simulink model "AA"  (R2021b)
settings: Solver=VariableStepAuto  StartTime=0.0  StopTime=50  RelTol=1e-3
values from neighbouring files (symbols this model uses):
  A = [ybb  yp+w0/u0 yr-1 g*ctt0/u0 ... (first row only)    [main.m]
  B = [0    ydr ... (first row only)    [main.m]
undefined symbols (not defined in the file or in its folder): C, D
settings Model: Creator=User  LastModifiedBy=User

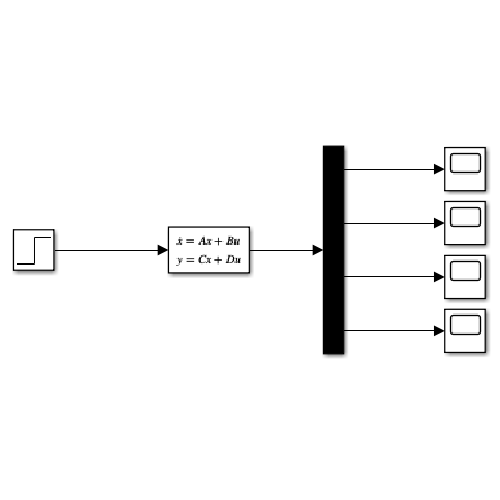
[thumbnail: Simulink's stored preview of the top-level diagram]
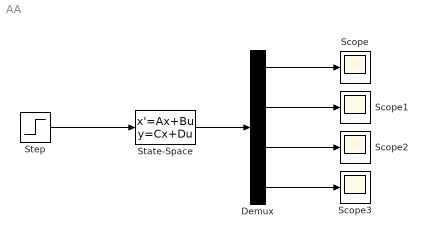
== system AA ==
  Demux : Demux
  Scope{,1..3} (4 alike) : Scope
  State-Space : StateSpace  A=A  B=B(:,1)  C=C  D=D(:,1)  InitialCondition=0
  Step : Step  Time=0  SampleTime=0
  wires:
  Step/1 -> State-Space/1
  State-Space/1 -> Demux/1
  Demux/1 -> Scope/1
  Demux/2 -> Scope1/1
  Demux/3 -> Scope2/1
  Demux/4 -> Scope3/1
